simulink model "getting_started_test_sfunction13a"  (Simulink 8.1)
settings: Solver=FixedStepDiscrete  StartTime=0.0  StopTime=15  FixedStep=0.3  RelTol=1e-3
settings Model: Creator=madwolf  LastModifiedBy=torstebo  SimulationMode=accelerator
settings DataIOCC: SignalLoggingSaveFormat=Dataset
settings OptimizationCC: ExpressionDepthLimit=128
settings DebuggingCC: FcnCallInpInsideContextMsg=EnableAllAsError  FrameProcessingCompatibilityMsg=error
settings SFSimCC: SimCustomHeaderCode="#include \"acado_solver_sfunction.h\""
settings RTWCC: TargetLang=C++
settings GRTTargetCC: CodeReplacementLibrary=C89/C90 (ANSI)  CombineOutputUpdateFcns=on  GRTInterface=off

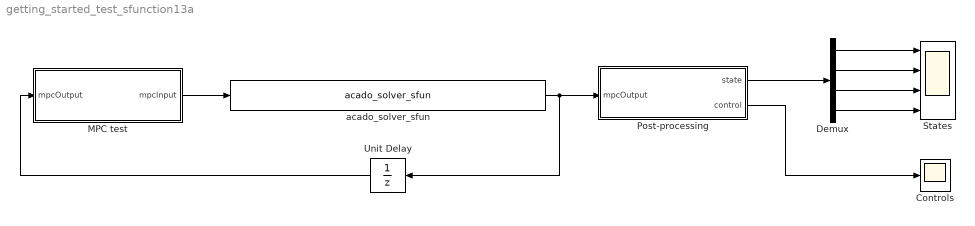
== system getting_started_test_sfunction13a ==
  Controls : Scope
      settings: TimeRange=auto  MaxDataPoints=5000  SaveToWorkspace=off  YMin=-1.16201  YMax=0.45812  SampleTime=-1
  Demux : Demux
  MPC test : MATLAB Function  TreatAsAtomicUnit=on
      settings: PermitHierarchicalResolution=ParametersOnly
  Post-processing : MATLAB Function  TreatAsAtomicUnit=on
      settings: PermitHierarchicalResolution=ParametersOnly
  States : Scope  NumInputPorts=4
      settings: TimeRange=auto  MaxDataPoints=5000  SaveToWorkspace=off  SaveName=ScopeData  YMin=-5~-5~-5~-5  YMax=5~5~5~5  SampleTime=-1
  Unit Delay : UnitDelay  SampleTime=-1
  acado_solver_sfun : S-Function  FunctionName=acado_solver_sfun  SFunctionDeploymentMode=off  EnableBusSupport=off  mask(Legacy Function){SFunctionSpec=acado_solver_wrapper(acadoinput u1[1], acadooutput y1[1]), ShowSpec=on}
      mask prompts: ShowSpec "Display function specification"
      mask help:
      | This block allows you to call the legacy functions specified by the following Legacy Code Tool definition:
      | def.SFunctionName = 'acado_solver_sfun';
      | def.OutputFcnSpec = 'acado_solver_wrapper(acadoinput u1[1], acadooutput y1[1])';
      | def.HeaderFiles = {'acado_common.h', 'acado_solver_sfunction.h'};
      | def.SourceFiles = {'qpoases/SRC/QProblem.cpp', 'qpoases/SRC/QProblemB.cpp', 'qpoases/SRC/Bounds.cpp', 'qpoases/SRC/Constraints.cpp', 'qpoases/SRC/SubjectTo.cpp', 'qpoases/SRC/Indexlist.cpp', 'qpoases/SRC/CyclingManager.cpp', 'qpoases/SRC/Utils.cpp', 'qpoases/SRC/MessageHandling.cpp', 'acado_solver.c', 'acado_integrator.c', 'acado_auxiliary_functions.c', 'acado_qpoases_interface.cpp', 'acado_solver_sfunction.c'};
      | def.IncPaths = {'qpoases', 'qpoases/INCLUDE', 'qpoases/SRC'};
      | def.Options.language = 'C++';
      mask Help: <p>This block was generated automatically by the Legacy Code Tool. For detailed help on this tool, call<a href="matlab:legacy_code('help')"> legacy_code('help')</a>.</p>
      mask Callback ShowSpec:
      | if strcmp(get_param(gcbh, 'ShowSpec'), 'on')
      |   set_param(gcbh, 'MaskDisplay', sprintf('fprintf(''%s'');', get_param(gcbh, 'SFunctionSpec')));
      | else
      |   set_param(gcbh, 'MaskDisplay', sprintf('fprintf(''%s'');', get_param(gcbh, 'FunctionName')));
      | end
      mask Display: fprintf('acado_solver_wrapper(acadoinput u1[1], acadooutput y1[1])');
  wires:
  MPC test/1(mpcInput) -> acado_solver_sfun/1
  Unit Delay/1 -> MPC test/1(mpcOutput)
  acado_solver_sfun/1 -> Post-processing/1(mpcOutput), Unit Delay/1
  Post-processing/2(control) -> Controls/1
  Demux/4 -> States/4
  Demux/3 -> States/3
  Demux/2 -> States/2
  Demux/1 -> States/1
  Post-processing/1(state) -> Demux/1

== matlab function Post-processing ==
  data: mpcOutput input Bus: ACADOoutput; state output double; control output double
function [state,control] = fcn(mpcOutput)
%#codegen

%% Setup dimensions
%  Those dimensions must match ones defined in the c++ code generator.
N   = 10;
NX  = 4;
NU  = 1;
NY  = 5;
NYN = 4;

%% Output data
state = mpcOutput.data.x(1, 1: NX);
control = mpcOutput.data.u(1, 1: NU);

== matlab function MPC test ==
  data: mpcInput output Bus: ACADOinput; mpcOutput input Bus: ACADOoutput
function mpcInput  = fcn(mpcOutput)
%#codegen

%% Setup dimensions
%  Those dimensions must match ones defined in the c++ code generator.
N   = 10;
NX  = 4;
NU  = 1;
NY  = 5;
NYN = 4;

%% Setup data structures

persistent firstRun
if isempty( firstRun )
    firstRun = 1;
end;

persistent input
if isempty ( input )
    % Simple running more
    input.control = int32( 0 );
    % Always use integration from the last node for shifting
    input.shifting = int32( 2 );
    % Initialization by a forward simulation.
    input.initialization = int32( 1 );
    
    %%% NOTE: All arrays are 1-D.
    input.data.x = zeros(1, (N + 1) * NX);
    input.data.u = zeros(1, N * NU);
    input.data.y = zeros(1, N * NY);
    input.data.yN = zeros(1, NYN);
    
    %%%  In case the weighting matrices are not fixed, add for example:
%     eye1 = eye( NY ) * 1;
%     eye5 = eye( NYN ) * 5;
%     
%     input.data.W = eye1(:)';
%     input.data.WN = eye5(:)';
    %%%
    
    input.data.x0 = zeros(1, NX);
end;

if firstRun == 1
    input.data.x0 = [2, 0, 0, 0];

    firstRun = 0;
else
    input.data.x = mpcOutput.data.x;
    input.data.u = mpcOutput.data.u;
    
    input.data.x0 = mpcOutput.data.x(1, NX + 1: 2 * NX);
end;

%% Output the data structures
mpcInput = input;
